simulink model "IM200HP_Test_Model_v2"  (Simulink 8.1)
settings: Solver=ode4  StartTime=0.0  StopTime=100  FixedStep=Ts  RelTol=1e-3
PostLoadFcn:
  | Ts=100e-6;
InitFcn:
  | Ts=100e-6;
libraries: powerlib x4, Load_lib x1, Motor_InductionMachine_lib x1
settings Model: Creator=ed12083  LastModifiedBy=re25624
settings DataIOCC: SignalLoggingSaveFormat=Dataset
settings OptimizationCC: ExpressionDepthLimit=128
settings DebuggingCC: FcnCallInpInsideContextMsg=EnableAllAsError
settings GRTTargetCC: CombineOutputUpdateFcns=on  GRTInterface=off

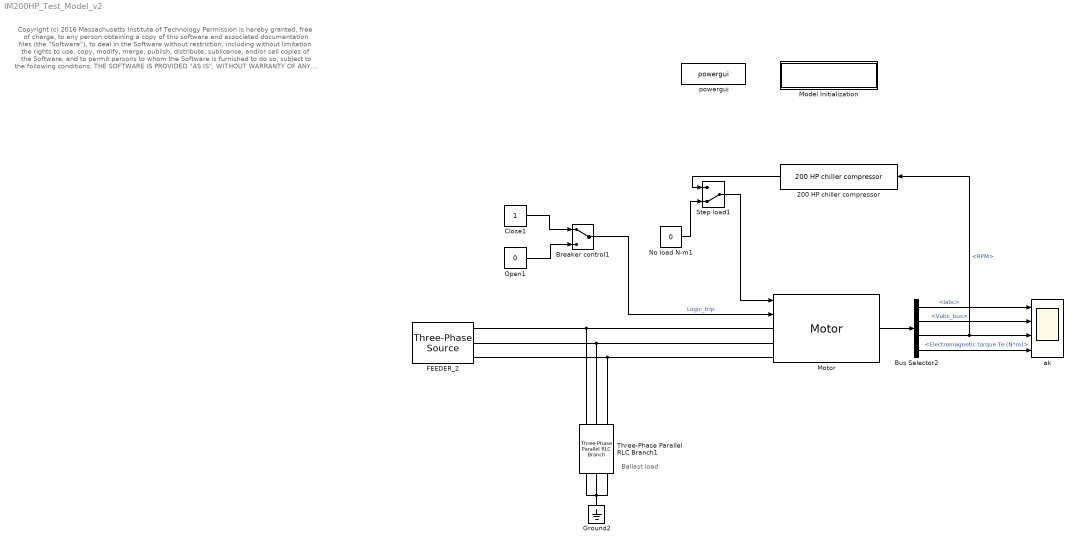
== system IM200HP_Test_Model_v2 ==
  note: Copyright (c) 2016 Massachusetts Institute of Technology
      | Permission is hereby granted, free of charge, to any person obtaining a copy of this software and associated documentation files (the "Software"), to deal
      | in the Software without restriction, including without limitation the rights to use, copy, modify, merge, publish, distribute, sublicense, and/or sell copies of the
      | Software, and to permit persons to whom the Software is furnished to do so, subject to the following conditions:
      |
      | THE SOFTWARE IS PROVIDED "AS IS", WITHOUT WARRANTY OF ANY KIND, EXPRESS OR IMPLIED, INCLUDING BUT NOT LIMITED TO THE
      | WARRANTIES OF MERCHANTABILITY, FITNESS FOR A PARTICULAR PURPOSE AND NONINFRINGEMENT. IN NO EVENT SHALL THE AUTHORS
      | OR COPYRIGHT HOLDERS BE LIABLE FOR ANY CLAIM, DAMAGES OR OTHER LIABILITY, WHETHER IN AN ACTION OF CONTRACT, TORT OR
      | OTHERWISE, ARISING FROM, OUT OF OR IN CONNECTION WITH THE SOFTWARE OR THE USE OR OTHER DEALINGS IN THE SOFTWARE.
  note: Ballast load
  200 HP chiller compressor : Load_lib/200 HP chiller compressor
  Breaker control1 : ManualSwitch
  Bus Selector2 : BusSelector  OutputSignals=Iabc,Vabc_bus,RPM,Electromagnetic torque Te (N*m)
  Close1 : Constant
  FEEDER_2 : powerlib/Electrical Sources/Three-Phase Source  Voltage=480  PhaseAngle=0  Frequency=60  InternalConnection=Yg  SpecifyImpedance=on  Resistance=0.8929  Inductance=16.58e-3  ShortCircuitLevel=375e6  BaseVoltage=480  XRratio=7.9  BusType=swing  Pref=0  Qref=0  Qmin=-inf  Qmax=inf
  Ground2 : powerlib/Elements/Ground  LConnTagsString=a
  Model Initialization : Subsystem  AncestorBlock=artemis/Tools /Misc/Model Initialization  mask(Model Functions){InitFcnX=Ts=100e-6;, prel=off, posl=on, inif=on, strf=off}
      mask prompts: InitFcnX "Initialisation"; prel "Preload Function"; posl "PostLoad Function"; inif "InitFcn"; strf "StartFcn"
      mask init:
      | currentBlock = gcb;
      | root = bdroot(currentBlock);
      | 
      | if ~strcmp(get_param(root,'BlockDiagramType'),'library')
      |     if prel==1
      |         set_param(root, 'PreLoadFcn', InitFcnX);
      |     else
      |         set_param(root, 'PreLoadFcn', '');
      |     end
      |     if inif==1
      |         set_param(root, 'InitFcn', InitFcnX);
      |     else
      |         set_param(root, 'InitFcn', '');
      |     end
      |     if strf==1
      |         set_param(root, 'StartFcn', InitFcnX);
      |     else
      |         set_param(root, 'StartFcn', '');
      |     end
      |     if posl==1
      |         set_param(root, 'PostLoadFcn', InitFcnX);
      |     else
      |         set_param(root, 'PostLoadFcn', '');
      |     end
      | end
      | 
      | pos = get_param(currentBlock, 'Position');
      | width = pos(3) - pos(1); height = pos(4) - pos(2);
      | txt = [ upper(root) '\n' '- InitFcn. . . . . '  get_param(root, 'InitFcn') ];
      settings: CopyFcn=set_param(gcb,'LinkStatus','inactive')
      mask Display: text(5, height*0.5, txt, 'horizontalAlignment', 'left', 'verticalAlignment', 'middle') ;
  Motor : Motor_InductionMachine_lib/Motor  Ts=Ts
  No load N-m1 : Constant  Value=0
  Open1 : Constant  Value=0
  Step load1 : ManualSwitch  CurrentSetting=0
  Three-Phase Parallel RLC Branch1 : powerlib/Elements/Three-Phase Parallel RLC Branch  LConnTagsString=A|B|C  RConnTagsString=A|B|C  BranchType=R  Resistance=1e6  Inductance=inf  Capacitance=inf  Measurements=None
  ak : Scope  NumInputPorts=4
      settings: ShowLegends=on  YMin=-1750~-450~0~-2000  YMax=1750~450~2000~3500  SaveName=ScopeData2
  powergui : powerlib/powergui  Priority=2  SimulationMode=Discrete  SolverType=Tustin  SampleTime=Ts  frequency=60  SPID=off  DisableSnubberDevices=off  DisableRonSwitches=off  DisableVfSwitches=off  SwTol=0  Interpol=off  DisplayEquations=off  frequencyindice=0  Pbase=100e6  ErrMax=1e-4  Iterations=50  UnitsV=kV  UnitsW=MW  FunctionMessages=off  echomessages=off  HookPort=off  EnableUseOfTLC=off  x0status=blocks  RestoreLinks=warning  ResistiveCurrentMeasurement=off  Frange=logspace(0,3,50)  Ylog=off  Xlog=off  ShowGrid=off  save=off  variable=ZData  structure=0  ZoomFFT=on  StartTime=0.0  cycles=2  DisplayStyle=off  fundamental=60  FreqAxis=off  MaxFrequency=1000  frequencyindicesteady=1  RmsSteady=1  display=off  Ts=0  methode=off
  wires:
  Motor/1 -> Bus Selector2/1
  Bus Selector2/3 -> 200 HP chiller compressor/1, ak/3  "<RPM>"
  Bus Selector2/1 -> ak/1  "<Iabc>"
  Bus Selector2/4 -> ak/4  "<Electromagnetic torque Te (N*m)>"
  Close1/1 -> Breaker control1/1
  Open1/1 -> Breaker control1/2
  Breaker control1/1 -> Motor/2  "Logic_trip"
  Bus Selector2/2 -> ak/2  "<Vabc_bus>"
  Step load1/1 -> Motor/1
  No load N-m1/1 -> Step load1/2
  200 HP chiller compressor/1 -> Step load1/1
  connections:
  FEEDER_2/RConn3 -- Motor/LConn3 -- Three-Phase Parallel RLC Branch1/RConn3
  FEEDER_2/RConn1 -- Motor/LConn1 -- Three-Phase Parallel RLC Branch1/RConn1
  FEEDER_2/RConn2 -- Motor/LConn2 -- Three-Phase Parallel RLC Branch1/RConn2
  Three-Phase Parallel RLC Branch1/LConn2 -- Three-Phase Parallel RLC Branch1/LConn1 -- Ground2/LConn1 -- Three-Phase Parallel RLC Branch1/LConn3

== system IM200HP_Test_Model_v2/Model Initialization ==
